simulink model "PosCtrl_tune"  (R2016b)
settings: Solver=FixedStepAuto  StartTime=0.0  StopTime=50  FixedStep=0.001  RelTol=1e-3
InitFcn:
  | Init_control;
undefined symbols (not defined in the file): DEG2RAD, DiscIntNeverNeededParam, Kd_PITCH_AgngleRate, Kd_ROLL_AgngleRate, Kd_YAW_AngleRate, Ki_PITCH_AgngleRate, Ki_ROLL_AgngleRate, Ki_YAW_AngleRate, Kp_PITCH_AgngleRate, Kp_PITCH_ANGLE, Kp_ROLL_AgngleRate, Kp_ROLL_ANGLE, Kp_YAW_AngleRate, Kpxp, Kpyp, Kpzp, Kvxd, Kvxi, Kvxp, Kvyd, Kvyi, Kvyp, Kvzd, Kvzi, Kvzp, MAX_CONTROL_ANGLE_PITCH, MAX_CONTROL_ANGLE_RATE_PITCH, MAX_CONTROL_ANGLE_RATE_ROLL, MAX_CONTROL_ANGLE_ROLL, MAX_CONTROL_VELOCITY_XY, MAX_CONTROL_VELOCITY_Z, MAX_MAN_THR, ModelInit_RPM, ModelParam_envGravityAcc, ModelParam_motorCr, ModelParam_motorJm, ModelParam_motorT, ModelParam_motorWb, ModelParam_rotorCm, ModelParam_rotorCt, ModelParam_uavCd, ModelParam_uavJ, ModelParam_uavMass, ModelParam_uavR, Saturation_I_ah, Saturation_I_az, Saturation_I_RP_Max, Saturation_I_RP_Min, Saturation_I_Y_Max, Saturation_I_Y_Min, THR_HOVER
libraries: simulink x6, aerolibutil x2, aerolibtransform2 x1
settings Model: Creator=dream  LastModifiedBy=Mr Wang
settings DebuggingCC: BusObjectLabelMismatch=error

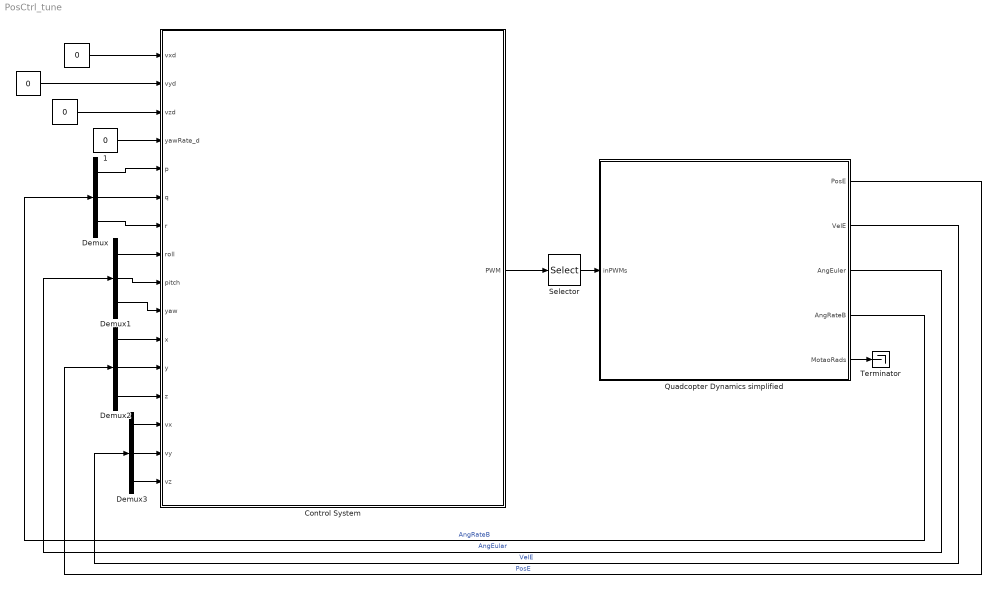
== system PosCtrl_tune ==
  "   " : Constant  Value=0  OutDataTypeStr=uint16
  "      " : Constant  Value=0  OutDataTypeStr=uint16
  "          " : Constant  Value=0  OutDataTypeStr=uint16
  "          1" : Constant  Value=0  OutDataTypeStr=uint16
  Control System : Subsystem
      mask Display: image('icon\pixhawk.png');
  Demux{,1..3} (4 alike) : Demux  Outputs=3
  "Quadcopter Dynamics simplified " : Subsystem
      mask Display: image('./icon/F450.png');
  Selector : Selector  InputPortWidth=8  IndexOptions=Index vector (dialog)  Indices=[1:4]  OutputSizes=1
  Terminator : Terminator
  wires:
  "Quadcopter Dynamics simplified "/1(PosE) -> Demux2/1  "PosE"
  "Quadcopter Dynamics simplified "/3(AngEuler) -> Demux1/1  "AngEular"
  "Quadcopter Dynamics simplified "/4(AngRateB) -> Demux/1  "AngRateB"
  Demux/1 -> Control System/5(p)
  Demux/2 -> Control System/6(q)
  Demux/3 -> Control System/7(r)
  Demux1/1 -> Control System/8(roll)
  Demux1/2 -> Control System/9(pitch)
  Demux1/3 -> Control System/10(yaw)
  Demux2/1 -> Control System/11(x)
  Demux2/2 -> Control System/12(y)
  Demux2/3 -> Control System/13(z)
  Demux3/1 -> Control System/14(vx)
  Demux3/2 -> Control System/15(vy)
  Demux3/3 -> Control System/16(vz)
  "Quadcopter Dynamics simplified "/2(VelE) -> Demux3/1  "VelE"
  "          "/1 -> Control System/3(vzd)
  "      "/1 -> Control System/2(vyd)
  "   "/1 -> Control System/1(vxd)
  "          1"/1 -> Control System/4(yawRate_d)
  Control System/1(PWM) -> Selector/1
  Selector/1 -> "Quadcopter Dynamics simplified "/1(inPWMs)
  "Quadcopter Dynamics simplified "/5(MotaoRads) -> Terminator/1

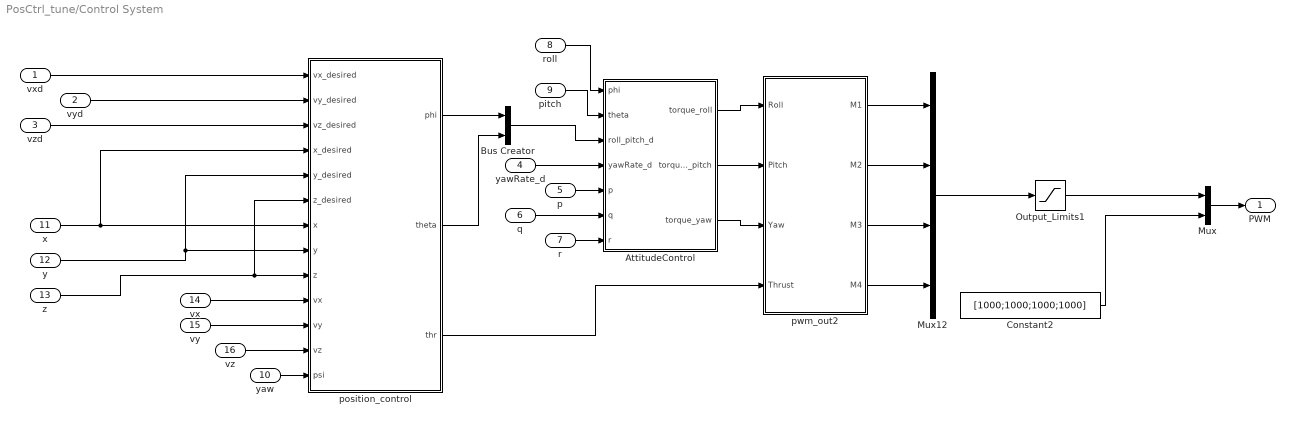
== system PosCtrl_tune/Control System ==
  vxd : Inport
  vyd : Inport  Port=2
  vzd : Inport  Port=3
  yawRate_d : Inport  Port=4
  p : Inport  Port=5  PortDimensions=1
  q : Inport  Port=6  PortDimensions=1
  r : Inport  Port=7  PortDimensions=1
  roll : Inport  Port=8  PortDimensions=1
  pitch : Inport  Port=9  PortDimensions=1
  yaw : Inport  Port=10  PortDimensions=1
  x : Inport  Port=11
  y : Inport  Port=12
  z : Inport  Port=13
  vx : Inport  Port=14
  vy : Inport  Port=15
  vz : Inport  Port=16
  AttitudeControl : Subsystem
  Bus Creator : BusCreator  Inputs=2
  Constant2 : Constant  Value=[1000;1000;1000;1000]
  Mux : Mux  Inputs=2
  Mux12 : Mux
  Output_Limits1 : Saturate  UpperLimit=2000  LowerLimit=1000
  position_control : Subsystem
  pwm_out2 : MATLAB Function  SystemSampleTime=0.004
  PWM : Outport  PortDimensions=8
  wires:
  Mux12/1 -> Output_Limits1/1
  AttitudeControl/2(torque_pitch) -> pwm_out2/2(Pitch)
  AttitudeControl/1(torque_roll) -> pwm_out2/1(Roll)
  pwm_out2/1(M1) -> Mux12/1
  pwm_out2/3(M3) -> Mux12/3
  pwm_out2/2(M2) -> Mux12/2
  AttitudeControl/3(torque_yaw) -> pwm_out2/3(Yaw)
  yawRate_d/1 -> AttitudeControl/4(yawRate_d)
  p/1 -> AttitudeControl/5(p)
  pwm_out2/4(M4) -> Mux12/4
  roll/1 -> AttitudeControl/1(phi)
  pitch/1 -> AttitudeControl/2(theta)
  position_control/1(phi) -> Bus Creator/1
  position_control/2(theta) -> Bus Creator/2
  Bus Creator/1 -> AttitudeControl/3(roll_pitch_d)
  position_control/3(thr) -> pwm_out2/4(Thrust)
  vxd/1 -> position_control/1(vx_desired)
  vyd/1 -> position_control/2(vy_desired)
  vzd/1 -> position_control/3(vz_desired)
  x/1 -> position_control/4(x_desired), position_control/7(x)
  y/1 -> position_control/5(y_desired), position_control/8(y)
  z/1 -> position_control/9(z), position_control/6(z_desired)
  vx/1 -> position_control/10(vx)
  vy/1 -> position_control/11(vy)
  vz/1 -> position_control/12(vz)
  yaw/1 -> position_control/13(psi)
  Constant2/1 -> Mux/2
  Output_Limits1/1 -> Mux/1
  Mux/1 -> PWM/1
  r/1 -> AttitudeControl/7(r)
  q/1 -> AttitudeControl/6(q)

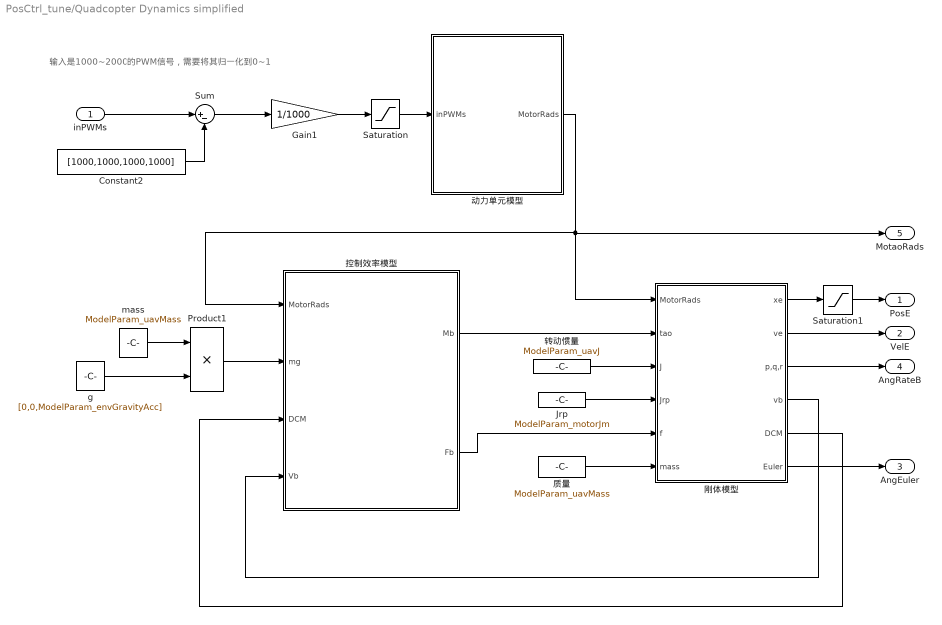
== system PosCtrl_tune/Quadcopter Dynamics simplified  ==
  note: 输入是1000~2000的PWM信号，需要将其归一化到0~1
  inPWMs : Inport
  Constant2 : Constant  Value=[1000,1000,1000,1000]
  Gain1 : Gain  Gain=1/1000
  Jrp : Constant  Value=ModelParam_motorJm
  Product1 : Product
  Saturation : Saturate  UpperLimit=1  LowerLimit=0
  Saturation1 : Saturate  UpperLimit=[inf,inf,0]  LowerLimit=[-inf,-inf,-inf]
  Sum : Sum  Inputs=|+-
  g : Constant  Value=[0,0,ModelParam_envGravityAcc]
  mass : Constant  Value=ModelParam_uavMass
  刚体模型 : Subsystem
  动力单元模型 : Subsystem
  控制效率模型 : Subsystem
  质量 : Constant  Value=ModelParam_uavMass
  转动惯量 : Constant  Value=ModelParam_uavJ
  PosE : Outport
  VelE : Outport  Port=2
  AngEuler : Outport  Port=3
  AngRateB : Outport  Port=4
  MotaoRads : Outport  Port=5
  wires:
  Saturation/1 -> 动力单元模型/1(inPWMs)
  刚体模型/3("p,q,r ") -> AngRateB/1
  Jrp/1 -> 刚体模型/4(Jrp)
  质量/1 -> 刚体模型/6(mass)
  mass/1 -> Product1/1
  刚体模型/5(DCM) -> 控制效率模型/3(DCM)
  刚体模型/1("xe ") -> Saturation1/1
  动力单元模型/1(MotorRads) -> 控制效率模型/1(MotorRads), 刚体模型/1(MotorRads), MotaoRads/1
  转动惯量/1 -> 刚体模型/3(J)
  Gain1/1 -> Saturation/1
  刚体模型/2(ve) -> VelE/1
  Sum/1 -> Gain1/1
  Product1/1 -> 控制效率模型/2(mg)
  刚体模型/4("vb ") -> 控制效率模型/4(Vb)
  Saturation1/1 -> PosE/1
  刚体模型/6(Euler) -> AngEuler/1
  控制效率模型/1(Mb) -> 刚体模型/2(tao)
  inPWMs/1 -> Sum/1
  控制效率模型/2(Fb) -> 刚体模型/5(f)
  Constant2/1 -> Sum/2
  g/1 -> Product1/2

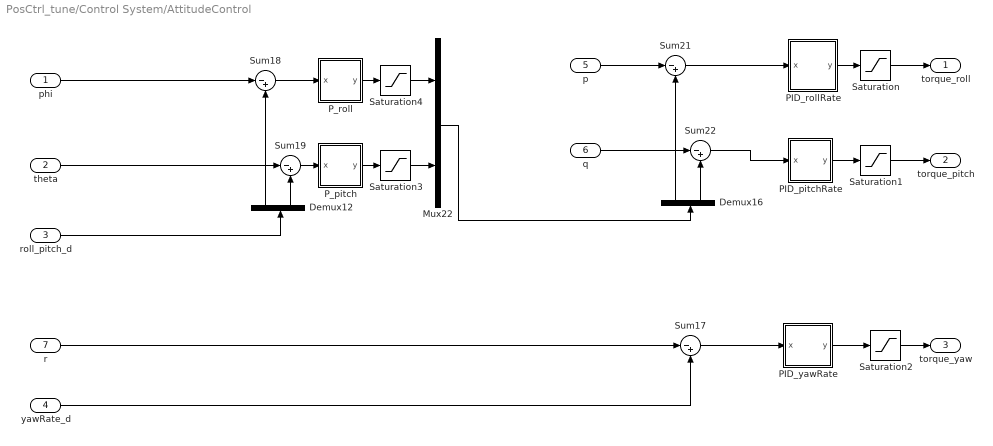
== system PosCtrl_tune/Control System/AttitudeControl ==
  phi : Inport
  theta : Inport  Port=2
  roll_pitch_d : Inport  Port=3
  yawRate_d : Inport  Port=4
  p : Inport  Port=5
  q : Inport  Port=6
  r : Inport  Port=7
  Demux12 : Demux  Outputs=2
  Demux16 : Demux  Outputs=2
  Mux22 : Mux  Inputs=2
  PID_pitchRate : Subsystem
  PID_rollRate : Subsystem
  PID_yawRate : Subsystem
  "P_pitch " : Subsystem
  "P_roll " : Subsystem
  Saturation : Saturate  UpperLimit=1  LowerLimit=-1
  Saturation1 : Saturate  UpperLimit=1  LowerLimit=-1
  Saturation2 : Saturate
  Saturation3 : Saturate  UpperLimit=MAX_CONTROL_ANGLE_RATE_PITCH  LowerLimit=-MAX_CONTROL_ANGLE_RATE_PITCH
  Saturation4 : Saturate  UpperLimit=MAX_CONTROL_ANGLE_RATE_ROLL  LowerLimit=-MAX_CONTROL_ANGLE_RATE_ROLL
  Sum{17..19,21..22} (5 alike) : Sum  Inputs=|-+
  torque_roll : Outport
  torque_pitch : Outport  Port=2
  torque_yaw : Outport  Port=3
  wires:
  r/1 -> Sum17/1
  Sum19/1 -> "P_pitch "/1(x)
  "P_pitch "/1(y) -> Saturation3/1
  "P_roll "/1(y) -> Saturation4/1
  roll_pitch_d/1 -> Demux12/1
  Demux12/1 -> Sum18/2
  Demux12/2 -> Sum19/2
  phi/1 -> Sum18/1
  theta/1 -> Sum19/1
  Sum18/1 -> "P_roll "/1(x)
  Sum22/1 -> PID_pitchRate/1(x)
  Sum17/1 -> PID_yawRate/1(x)
  p/1 -> Sum21/1
  q/1 -> Sum22/1
  Sum21/1 -> PID_rollRate/1(x)
  Demux16/1 -> Sum21/2
  PID_pitchRate/1(y) -> Saturation1/1
  PID_rollRate/1(y) -> Saturation/1
  PID_yawRate/1(y) -> Saturation2/1
  yawRate_d/1 -> Sum17/2
  Saturation/1 -> torque_roll/1
  Saturation1/1 -> torque_pitch/1
  Saturation2/1 -> torque_yaw/1
  Mux22/1 -> Demux16/1
  Saturation4/1 -> Mux22/1
  Saturation3/1 -> Mux22/2
  Demux16/2 -> Sum22/2

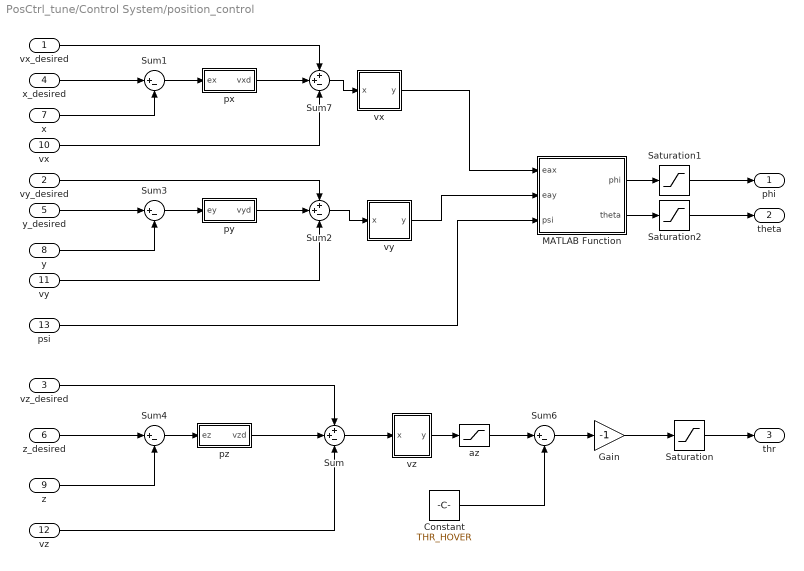
== system PosCtrl_tune/Control System/position_control ==
  vx_desired : Inport
  vy_desired : Inport  Port=2
  vz_desired : Inport  Port=3
  x_desired : Inport  Port=4
  y_desired : Inport  Port=5
  z_desired : Inport  Port=6
  x : Inport  Port=7
  y : Inport  Port=8
  z : Inport  Port=9
  vx : Inport  Port=10
  vy : Inport  Port=11
  vz : Inport  Port=12
  psi : Inport  Port=13
  Constant : Constant  Value=THR_HOVER
  Gain : Gain  Gain=-1
  MATLAB Function : MATLAB Function  TreatAsAtomicUnit=on
  Saturation : Saturate  UpperLimit=MAX_MAN_THR  LowerLimit=0
  Saturation1 : Saturate  UpperLimit=MAX_CONTROL_ANGLE_ROLL*DEG2RAD  LowerLimit=-MAX_CONTROL_ANGLE_ROLL*DEG2RAD
  Saturation2 : Saturate  UpperLimit=MAX_CONTROL_ANGLE_PITCH*DEG2RAD  LowerLimit=-MAX_CONTROL_ANGLE_PITCH*DEG2RAD
  Sum : Sum  Inputs=++-
  Sum{1,3..4,6} (4 alike) : Sum  Inputs=|+-
  Sum2 : Sum  Inputs=++-
  Sum7 : Sum  Inputs=++-
  az : Saturate  UpperLimit=0.4  LowerLimit=-0.4
  px : Subsystem
  py : Subsystem
  pz : Subsystem
  "vx " : Subsystem
  "vy " : Subsystem
  "vz " : Subsystem
  phi : Outport
  theta : Outport  Port=2
  thr : Outport  Port=3
  wires:
  Saturation/1 -> thr/1
  Gain/1 -> Saturation/1
  Sum6/1 -> Gain/1
  "vz "/1(y) -> az/1
  Sum4/1 -> pz/1(ez)
  z/1 -> Sum4/2
  Constant/1 -> Sum6/2
  Sum/1 -> "vz "/1(x)
  vz/1 -> Sum/3
  x/1 -> Sum1/2
  y/1 -> Sum3/2
  Sum3/1 -> py/1(ey)
  y_desired/1 -> Sum3/1
  vy/1 -> Sum2/3
  Sum2/1 -> "vy "/1(x)
  Sum7/1 -> "vx "/1(x)
  Sum1/1 -> px/1(ex)
  vy_desired/1 -> Sum2/1
  pz/1(vzd) -> Sum/2
  z_desired/1 -> Sum4/1
  vz_desired/1 -> Sum/1
  Saturation1/1 -> phi/1
  Saturation2/1 -> theta/1
  psi/1 -> MATLAB Function/3(psi)
  py/1(vyd) -> Sum2/2
  MATLAB Function/1(phi) -> Saturation1/1
  MATLAB Function/2(theta) -> Saturation2/1
  "vx "/1(y) -> MATLAB Function/1(eax)
  "vy "/1(y) -> MATLAB Function/2(eay)
  az/1 -> Sum6/1
  vx_desired/1 -> Sum7/1
  x_desired/1 -> Sum1/1
  vx/1 -> Sum7/3
  px/1(vxd) -> Sum7/2

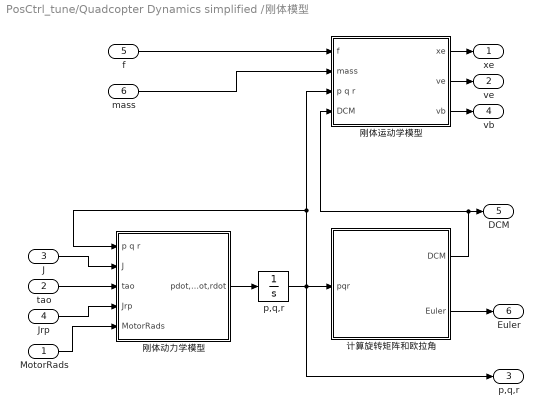
== system PosCtrl_tune/Quadcopter Dynamics simplified /刚体模型 ==
  MotorRads : Inport
  tao : Inport  Port=2
  J : Inport  Port=3
  Jrp : Inport  Port=4
  f : Inport  Port=5
  mass : Inport  Port=6
  p,q,r : Integrator
  刚体动力学模型 : Subsystem
  刚体运动学模型 : Subsystem
  计算旋转矩阵和欧拉角 : Subsystem
  "xe " : Outport
  ve : Outport  Port=2
  "p,q,r " : Outport  Port=3
  "vb " : Outport  Port=4
  DCM : Outport  Port=5
  Euler : Outport  Port=6
  wires:
  刚体运动学模型/3("vb ") -> "vb "/1
  p,q,r/1 -> 计算旋转矩阵和欧拉角/1(pqr), "p,q,r "/1, 刚体动力学模型/1(p q r), 刚体运动学模型/3(p q r)
  刚体运动学模型/2(ve) -> ve/1
  刚体运动学模型/1("xe ") -> "xe "/1
  mass/1 -> 刚体运动学模型/2(mass)
  f/1 -> 刚体运动学模型/1(f)
  计算旋转矩阵和欧拉角/2(Euler) -> Euler/1
  计算旋转矩阵和欧拉角/1(DCM) -> 刚体运动学模型/4(DCM), DCM/1
  刚体动力学模型/1(pdot,qdot,rdot) -> p,q,r/1
  MotorRads/1 -> 刚体动力学模型/5(MotorRads)
  Jrp/1 -> 刚体动力学模型/4(Jrp)
  tao/1 -> 刚体动力学模型/3(tao)
  J/1 -> 刚体动力学模型/2(J)

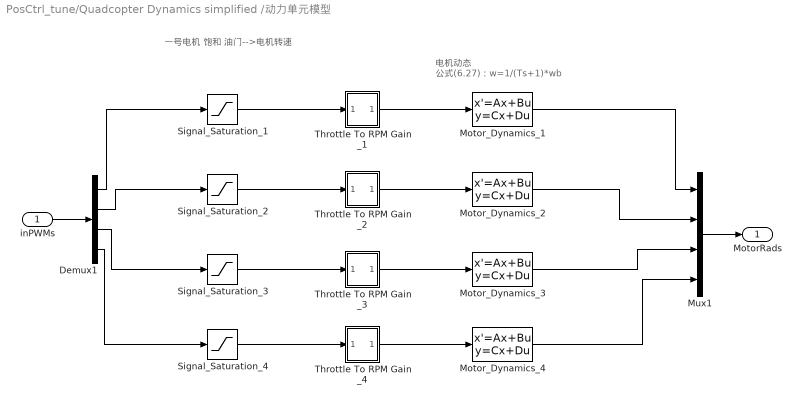
== system PosCtrl_tune/Quadcopter Dynamics simplified /动力单元模型 ==
  note: 电机动态
      | 公式(6.27)：w=1/(Ts+1)*wb
  note: 一号电机
      |
      |              饱和                             油门-->电机转速
  inPWMs : Inport
  Demux1 : Demux
  Motor_Dynamics_{1..4} (4 alike) : StateSpace  A=-1/ModelParam_motorT  C=1/ModelParam_motorT  D=0  X0=ModelInit_RPM*ModelParam_motorT
  Mux1 : Mux
  Signal_Saturation_{1..4} (4 alike) : Saturate  UpperLimit=1  LowerLimit=0
  Throttle To RPM Gain _1 : Subsystem
  Throttle To RPM Gain _2 : Subsystem
  Throttle To RPM Gain _3 : Subsystem
  Throttle To RPM Gain _4 : Subsystem
  MotorRads : Outport
  wires:
  Throttle To RPM Gain _4/1(Out5) -> Motor_Dynamics_4/1
  Signal_Saturation_4/1 -> Throttle To RPM Gain _4/1(In5)
  Signal_Saturation_3/1 -> Throttle To RPM Gain _3/1(In5)
  Signal_Saturation_2/1 -> Throttle To RPM Gain _2/1(In5)
  Motor_Dynamics_4/1 -> Mux1/4
  Motor_Dynamics_3/1 -> Mux1/3
  Motor_Dynamics_2/1 -> Mux1/2
  Motor_Dynamics_1/1 -> Mux1/1
  Signal_Saturation_1/1 -> Throttle To RPM Gain _1/1(In5)
  Mux1/1 -> MotorRads/1
  Throttle To RPM Gain _3/1(Out5) -> Motor_Dynamics_3/1
  Throttle To RPM Gain _2/1(Out5) -> Motor_Dynamics_2/1
  Throttle To RPM Gain _1/1(Out5) -> Motor_Dynamics_1/1
  inPWMs/1 -> Demux1/1
  Demux1/4 -> Signal_Saturation_4/1
  Demux1/3 -> Signal_Saturation_3/1
  Demux1/2 -> Signal_Saturation_2/1
  Demux1/1 -> Signal_Saturation_1/1

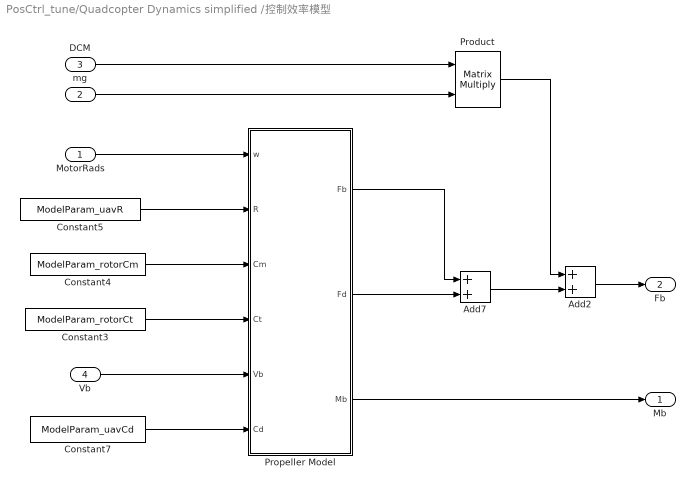
== system PosCtrl_tune/Quadcopter Dynamics simplified /控制效率模型 ==
  MotorRads : Inport
  mg : Inport  Port=2
  DCM : Inport  Port=3
  Vb : Inport  Port=4
  Add2 : Sum
  Add7 : Sum
  Constant3 : Constant  Value=ModelParam_rotorCt
  Constant4 : Constant  Value=ModelParam_rotorCm
  Constant5 : Constant  Value=ModelParam_uavR
  Constant7 : Constant  Value=ModelParam_uavCd
  Product : Product  Multiplication=Matrix(*)
  Propeller Model : MATLAB Function  TreatAsAtomicUnit=on
  Mb : Outport
  Fb : Outport  Port=2
  wires:
  Propeller Model/3(Mb) -> Mb/1
  Add2/1 -> Fb/1
  Constant3/1 -> Propeller Model/4(Ct)
  Propeller Model/2(Fd) -> Add7/2
  Add7/1 -> Add2/2
  Propeller Model/1(Fb) -> Add7/1
  Product/1 -> Add2/1
  mg/1 -> Product/2
  DCM/1 -> Product/1
  Constant7/1 -> Propeller Model/6(Cd)
  Vb/1 -> Propeller Model/5(Vb)
  Constant5/1 -> Propeller Model/2(R)
  Constant4/1 -> Propeller Model/3(Cm)
  MotorRads/1 -> Propeller Model/1(w)

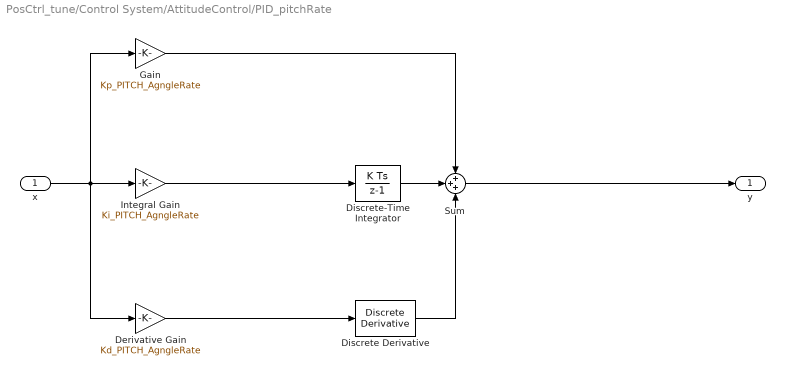
== system PosCtrl_tune/Control System/AttitudeControl/PID_pitchRate ==
  x : Inport
  Derivative Gain : Gain  DisableCoverage=on  Gain=Kd_PITCH_AgngleRate  ParamMin=-100  ParamMax=100  OutMin=-100  OutMax=100
  Discrete Derivative : simulink/Discrete/Discrete Derivative  gainval=1.0  ICPrevScaledInput=0.0  OutMin=[]  OutMax=[]  OutDataType=fixdt(1, 16)  OutScaling=2^-10  DoSatur=off
  Discrete-Time Integrator : DiscreteIntegrator  InitialConditionSetting=State (most efficient)  SampleTime=-1  LimitOutput=on  UpperSaturationLimit=Saturation_I_RP_Max  LowerSaturationLimit=Saturation_I_RP_Min  ICPrevOutput=DiscIntNeverNeededParam  ICPrevScaledInput=DiscIntNeverNeededParam
  Gain : Gain  Gain=Kp_PITCH_AgngleRate
  Integral Gain : Gain  DisableCoverage=on  Gain=Ki_PITCH_AgngleRate
  Sum : Sum  Inputs=+++
  y : Outport  InitialOutput=0
  wires:
  Discrete-Time Integrator/1 -> Sum/2
  Discrete Derivative/1 -> Sum/3
  Sum/1 -> y/1
  Gain/1 -> Sum/1
  Derivative Gain/1 -> Discrete Derivative/1
  Integral Gain/1 -> Discrete-Time Integrator/1
  x/1 -> Derivative Gain/1, Integral Gain/1, Gain/1

== system PosCtrl_tune/Control System/AttitudeControl/PID_rollRate ==
  x : Inport
  Derivative Gain : Gain  DisableCoverage=on  Gain=Kd_ROLL_AgngleRate  ParamMin=-100  ParamMax=100  OutMin=-100  OutMax=100
  Discrete Derivative : simulink/Discrete/Discrete Derivative  gainval=1.0  ICPrevScaledInput=0.0  OutMin=[]  OutMax=[]  OutDataType=fixdt(1, 16)  OutScaling=2^-10  DoSatur=off
  Discrete-Time Integrator : DiscreteIntegrator  InitialConditionSetting=State (most efficient)  SampleTime=-1  LimitOutput=on  UpperSaturationLimit=Saturation_I_RP_Max  LowerSaturationLimit=Saturation_I_RP_Min  ICPrevOutput=DiscIntNeverNeededParam  ICPrevScaledInput=DiscIntNeverNeededParam
  Gain : Gain  Gain=Kp_ROLL_AgngleRate
  Integral Gain : Gain  DisableCoverage=on  Gain=Ki_ROLL_AgngleRate
  Sum : Sum  Inputs=+++
  y : Outport  InitialOutput=0
  wires:
  x/1 -> Gain/1, Integral Gain/1, Derivative Gain/1
  Integral Gain/1 -> Discrete-Time Integrator/1
  Derivative Gain/1 -> Discrete Derivative/1
  Gain/1 -> Sum/1
  Sum/1 -> y/1
  Discrete Derivative/1 -> Sum/3
  Discrete-Time Integrator/1 -> Sum/2

== system PosCtrl_tune/Control System/AttitudeControl/PID_yawRate ==
  x : Inport
  Derivative Gain : Gain  DisableCoverage=on  Gain=Kd_YAW_AngleRate  ParamMin=-100  ParamMax=100  OutMin=-100  OutMax=100
  Discrete Derivative : simulink/Discrete/Discrete Derivative  gainval=1.0  ICPrevScaledInput=0.0  OutMin=[]  OutMax=[]  OutDataType=fixdt(1, 16)  OutScaling=2^-10  DoSatur=off
  Discrete-Time Integrator : DiscreteIntegrator  InitialConditionSetting=State (most efficient)  SampleTime=-1  LimitOutput=on  UpperSaturationLimit=Saturation_I_Y_Max  LowerSaturationLimit=Saturation_I_Y_Min  ICPrevOutput=DiscIntNeverNeededParam  ICPrevScaledInput=DiscIntNeverNeededParam
  Gain : Gain  Gain=Kp_YAW_AngleRate
  Integral Gain : Gain  DisableCoverage=on  Gain=Ki_YAW_AngleRate
  Sum : Sum  Inputs=+++
  y : Outport  InitialOutput=0
  wires:
  x/1 -> Gain/1, Integral Gain/1, Derivative Gain/1
  Integral Gain/1 -> Discrete-Time Integrator/1
  Derivative Gain/1 -> Discrete Derivative/1
  Gain/1 -> Sum/1
  Sum/1 -> y/1
  Discrete Derivative/1 -> Sum/3
  Discrete-Time Integrator/1 -> Sum/2

== system PosCtrl_tune/Control System/AttitudeControl/P_pitch  ==
  x : Inport
  Gain : Gain  Gain=Kp_PITCH_ANGLE
  y : Outport  InitialOutput=0
  wires:
  x/1 -> Gain/1
  Gain/1 -> y/1

== system PosCtrl_tune/Control System/AttitudeControl/P_roll  ==
  x : Inport
  Gain : Gain  Gain=Kp_ROLL_ANGLE
  y : Outport  InitialOutput=0
  wires:
  Gain/1 -> y/1
  x/1 -> Gain/1

== system PosCtrl_tune/Control System/position_control/px ==
  ex : Inport
  Gain1 : Gain  Gain=Kpxp
  Saturation3 : Saturate  UpperLimit=MAX_CONTROL_VELOCITY_XY  LowerLimit=-MAX_CONTROL_VELOCITY_XY
  vxd : Outport
  wires:
  ex/1 -> Gain1/1
  Saturation3/1 -> vxd/1
  Gain1/1 -> Saturation3/1

== system PosCtrl_tune/Control System/position_control/py ==
  ey : Inport
  Gain1 : Gain  Gain=Kpyp
  Saturation3 : Saturate  UpperLimit=MAX_CONTROL_VELOCITY_XY  LowerLimit=-MAX_CONTROL_VELOCITY_XY
  vyd : Outport
  wires:
  Gain1/1 -> Saturation3/1
  Saturation3/1 -> vyd/1
  ey/1 -> Gain1/1

== system PosCtrl_tune/Control System/position_control/pz ==
  ez : Inport
  Gain1 : Gain  Gain=Kpzp
  Saturation3 : Saturate  UpperLimit=MAX_CONTROL_VELOCITY_Z  LowerLimit=-MAX_CONTROL_VELOCITY_Z
  vzd : Outport
  wires:
  ez/1 -> Gain1/1
  Saturation3/1 -> vzd/1
  Gain1/1 -> Saturation3/1

== system PosCtrl_tune/Control System/position_control/vx  ==
  x : Inport
  Derivative Gain : Gain  DisableCoverage=on  Gain=Kvxd
  Discrete Derivative : simulink/Discrete/Discrete Derivative  gainval=1.0  ICPrevScaledInput=0.0  OutMin=[]  OutMax=[]  OutDataType=fixdt(1, 16)  OutScaling=2^-10  DoSatur=off
  Discrete-Time Integrator : DiscreteIntegrator  InitialConditionSetting=State (most efficient)  SampleTime=-1  LimitOutput=on  UpperSaturationLimit=Saturation_I_ah  LowerSaturationLimit=-Saturation_I_ah  ICPrevOutput=DiscIntNeverNeededParam  ICPrevScaledInput=DiscIntNeverNeededParam
  Gain : Gain  Gain=Kvxp
  Integral Gain : Gain  DisableCoverage=on  Gain=Kvxi
  Sum : Sum  Inputs=+++
  y : Outport  InitialOutput=0
  wires:
  x/1 -> Gain/1, Integral Gain/1, Derivative Gain/1
  Integral Gain/1 -> Discrete-Time Integrator/1
  Derivative Gain/1 -> Discrete Derivative/1
  Gain/1 -> Sum/1
  Sum/1 -> y/1
  Discrete Derivative/1 -> Sum/3
  Discrete-Time Integrator/1 -> Sum/2

== system PosCtrl_tune/Control System/position_control/vy  ==
  x : Inport
  Derivative Gain : Gain  DisableCoverage=on  Gain=Kvyd
  Discrete Derivative : simulink/Discrete/Discrete Derivative  gainval=1.0  ICPrevScaledInput=0.0  OutMin=-5  OutMax=5  OutDataType=fixdt(1, 16)  OutScaling=2^-10  DoSatur=off
  Discrete-Time Integrator : DiscreteIntegrator  InitialConditionSetting=State (most efficient)  SampleTime=-1  LimitOutput=on  UpperSaturationLimit=Saturation_I_ah  LowerSaturationLimit=-Saturation_I_ah  ICPrevOutput=DiscIntNeverNeededParam  ICPrevScaledInput=DiscIntNeverNeededParam
  Gain : Gain  Gain=Kvyp
  Integral Gain : Gain  DisableCoverage=on  Gain=Kvyi
  Sum : Sum  Inputs=+++  OutMin=-5  OutMax=5
  y : Outport  InitialOutput=0
  wires:
  x/1 -> Gain/1, Integral Gain/1, Derivative Gain/1
  Integral Gain/1 -> Discrete-Time Integrator/1
  Derivative Gain/1 -> Discrete Derivative/1
  Gain/1 -> Sum/1
  Sum/1 -> y/1
  Discrete Derivative/1 -> Sum/3
  Discrete-Time Integrator/1 -> Sum/2

== system PosCtrl_tune/Control System/position_control/vz  ==
  x : Inport
  Derivative Gain : Gain  DisableCoverage=on  Gain=Kvzd
  Discrete Derivative : simulink/Discrete/Discrete Derivative  gainval=1.0  ICPrevScaledInput=0.0  OutMin=[]  OutMax=[]  OutDataType=fixdt(1, 16)  OutScaling=2^-10  DoSatur=off
  Discrete-Time Integrator : DiscreteIntegrator  InitialConditionSetting=State (most efficient)  SampleTime=-1  LimitOutput=on  UpperSaturationLimit=Saturation_I_az  LowerSaturationLimit=-Saturation_I_az  ICPrevOutput=DiscIntNeverNeededParam  ICPrevScaledInput=DiscIntNeverNeededParam
  Gain : Gain  Gain=Kvzp
  Integral Gain : Gain  DisableCoverage=on  Gain=Kvzi
  Sum : Sum  Inputs=+++
  y : Outport  InitialOutput=0
  wires:
  Discrete-Time Integrator/1 -> Sum/2
  Discrete Derivative/1 -> Sum/3
  Sum/1 -> y/1
  Gain/1 -> Sum/1
  Derivative Gain/1 -> Discrete Derivative/1
  Integral Gain/1 -> Discrete-Time Integrator/1
  x/1 -> Derivative Gain/1, Integral Gain/1, Gain/1

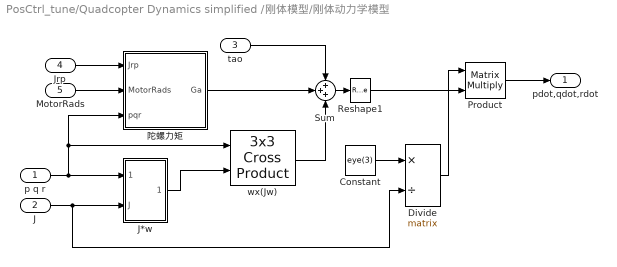
== system PosCtrl_tune/Quadcopter Dynamics simplified /刚体模型/刚体动力学模型 ==
  p q r : Inport
  J : Inport  Port=2
  tao : Inport  Port=3
  Jrp : Inport  Port=4
  MotorRads : Inport  Port=5
  Constant : Constant  Value=eye(3)
  Divide : Product  Inputs=*/  Multiplication=Matrix(*)
  J*w : Subsystem
  Product : Product  Multiplication=Matrix(*)
  Reshape1 : Reshape  OutputDimensionality=Column vector (2-D)
  Sum : Sum  Inputs=3
  wx(Jw) : aerolibutil/3x3 Cross Product
  陀螺力矩 : MATLAB Function  TreatAsAtomicUnit=on
  pdot,qdot,rdot : Outport
  wires:
  Product/1 -> pdot,qdot,rdot/1
  Reshape1/1 -> Product/2
  Constant/1 -> Divide/1
  陀螺力矩/1(Ga) -> Sum/2
  Divide/1 -> Product/1
  Sum/1 -> Reshape1/1
  J/1 -> Divide/2, J*w/2(J)
  p q r/1 -> J*w/1(p q r), 陀螺力矩/3(pqr), wx(Jw)/1
  J*w/1("J*w ") -> wx(Jw)/2
  tao/1 -> Sum/1
  Jrp/1 -> 陀螺力矩/1(Jrp)
  MotorRads/1 -> 陀螺力矩/2(MotorRads)
  wx(Jw)/1 -> Sum/3

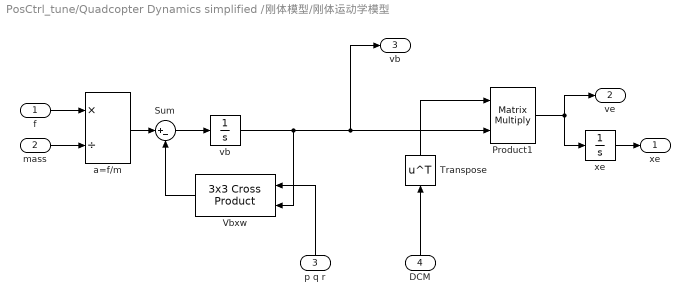
== system PosCtrl_tune/Quadcopter Dynamics simplified /刚体模型/刚体运动学模型 ==
  f : Inport
  mass : Inport  Port=2
  p q r : Inport  Port=3
  DCM : Inport  Port=4
  Product1 : Product  Multiplication=Matrix(*)
  Sum : Sum  Inputs=|+-
  Transpose : Math  Operator=transpose  SaturateOnIntegerOverflow=on
  Vbxw : aerolibutil/3x3 Cross Product
  a=f/m : Product  Inputs=*/
  vb : Integrator
  xe : Integrator
  "xe " : Outport
  ve : Outport  Port=2
  "vb " : Outport  Port=3
  wires:
  vb/1 -> Product1/2, "vb "/1, Vbxw/2
  a=f/m/1 -> Sum/1
  Sum/1 -> vb/1
  xe/1 -> "xe "/1
  Product1/1 -> xe/1, ve/1
  Transpose/1 -> Product1/1
  mass/1 -> a=f/m/2
  Vbxw/1 -> Sum/2
  f/1 -> a=f/m/1
  p q r/1 -> Vbxw/1
  DCM/1 -> Transpose/1

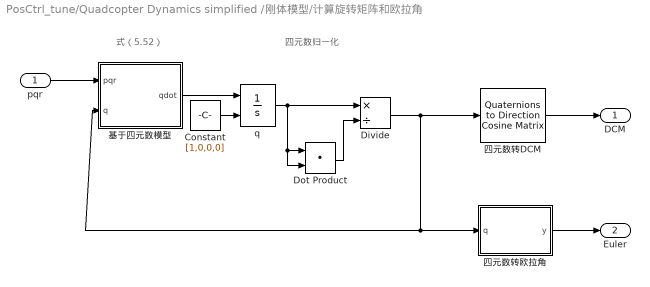
== system PosCtrl_tune/Quadcopter Dynamics simplified /刚体模型/计算旋转矩阵和欧拉角 ==
  note: 式（5.52）
  note: 四元数归一化
  pqr : Inport
  Constant : Constant  Value=[1,0,0,0]
  Divide : Product  Inputs=*/
  Dot Product : DotProduct  InputSameDT=on  OutDataTypeStr=Inherit: Inherit via internal rule
  q : Integrator  InitialConditionSource=external
  四元数转DCM : aerolibtransform2/Quaternions to  Direction Cosine Matrix
  四元数转欧拉角 : MATLAB Function
  基于四元数模型 : MATLAB Function  TreatAsAtomicUnit=on
  DCM : Outport
  Euler : Outport  Port=2
  wires:
  四元数转欧拉角/1(y) -> Euler/1
  Divide/1 -> 四元数转DCM/1, 基于四元数模型/2(q), 四元数转欧拉角/1(q)
  Dot Product/1 -> Divide/2
  四元数转DCM/1 -> DCM/1
  pqr/1 -> 基于四元数模型/1(pqr)
  q/1 -> Dot Product/1, Dot Product/2, Divide/1
  基于四元数模型/1(qdot) -> q/1
  Constant/1 -> q/2

== system PosCtrl_tune/Quadcopter Dynamics simplified /动力单元模型/Throttle To RPM Gain _1 ==
  In5 : Inport
  Constant : Constant  Value=ModelParam_motorWb
  Gain : Gain  Gain=ModelParam_motorCr
  Sum1 : Sum  Inputs=++|
  Out5 : Outport
  wires:
  Constant/1 -> Sum1/1
  Gain/1 -> Sum1/2
  In5/1 -> Gain/1
  Sum1/1 -> Out5/1

== system PosCtrl_tune/Quadcopter Dynamics simplified /动力单元模型/Throttle To RPM Gain _2 ==
  In5 : Inport
  Constant : Constant  Value=ModelParam_motorWb
  Gain : Gain  Gain=ModelParam_motorCr
  Sum1 : Sum  Inputs=++|
  Out5 : Outport
  wires:
  Sum1/1 -> Out5/1
  In5/1 -> Gain/1
  Gain/1 -> Sum1/2
  Constant/1 -> Sum1/1

== system PosCtrl_tune/Quadcopter Dynamics simplified /动力单元模型/Throttle To RPM Gain _3 ==
  In5 : Inport
  Constant : Constant  Value=ModelParam_motorWb
  Gain : Gain  Gain=ModelParam_motorCr
  Sum1 : Sum  Inputs=++|
  Out5 : Outport
  wires:
  Constant/1 -> Sum1/1
  Gain/1 -> Sum1/2
  In5/1 -> Gain/1
  Sum1/1 -> Out5/1

== system PosCtrl_tune/Quadcopter Dynamics simplified /动力单元模型/Throttle To RPM Gain _4 ==
  In5 : Inport
  Constant : Constant  Value=ModelParam_motorWb
  Gain : Gain  Gain=ModelParam_motorCr
  Sum1 : Sum  Inputs=++|
  Out5 : Outport
  wires:
  Sum1/1 -> Out5/1
  In5/1 -> Gain/1
  Gain/1 -> Sum1/2
  Constant/1 -> Sum1/1

== system PosCtrl_tune/Quadcopter Dynamics simplified /刚体模型/刚体动力学模型/J*w ==
  p q r : Inport
  J : Inport  Port=2
  J*w : Product  Multiplication=Matrix(*)
  "J*w " : Outport
  wires:
  J*w/1 -> "J*w "/1
  J/1 -> J*w/1
  p q r/1 -> J*w/2

== matlab function PosCtrl_tune/Control System/position_control/MATLAB Function ==
  data: eax input; eay input; psi input; phi output; theta output
function [phi,theta] = fcn(eax,eay,psi)
g=9.8;
phi = (-sin(psi)*eax + cos(psi)*eay)/g;
theta = (-cos(psi)*eax-sin(psi)*eay)/g;

== matlab function PosCtrl_tune/Control System/pwm_out2 ==
  data: Roll input; M1 output; Pitch input; Yaw input; Thrust input; M2 output; M3 output; M4 output
function [M1, M2, M3, M4] = motor_mixer(Roll, Pitch, Yaw, Thrust)
%quadrotorX
%3     1
%  \ /
%  / \
%2     4

idle_PWM = 1000;
scale = 1000;

M1 = (Thrust - Roll + Pitch + Yaw) * scale + idle_PWM;
M2 = (Thrust + Roll - Pitch + Yaw) * scale + idle_PWM;
M3 = (Thrust + Roll + Pitch - Yaw) * scale + idle_PWM;
M4 = (Thrust - Roll - Pitch - Yaw) * scale + idle_PWM;

== matlab function PosCtrl_tune/Quadcopter Dynamics simplified /刚体模型/刚体动力学模型/陀螺力矩 ==
  data: Jrp input; MotorRads input; pqr input; Ga output
function Ga = fcn(Jrp,MotorRads,pqr)
Ga=zeros(3,1);
Ga(1)=Jrp*pqr(2)*(-MotorRads(1)-MotorRads(2)+MotorRads(3)+MotorRads(4));
Ga(2)=Jrp*pqr(1)*( MotorRads(1)+MotorRads(2)-MotorRads(3)-MotorRads(4));

== matlab function PosCtrl_tune/Quadcopter Dynamics simplified /刚体模型/计算旋转矩阵和欧拉角/四元数转欧拉角 ==
  data: q input; y output
function y = fcn(q)
Rbe = [q(1)*q(1) + q(2)*q(2) - q(3)*q(3) - q(4)*q(4), 2*(q(2)*q(3) - q(1)*q(4)), 2*(q(2)*q(4) + q(1)*q(3))
       2*(q(2)*q(3) + q(1)*q(4)), q(1)*q(1) - q(2)*q(2) + q(3)*q(3) - q(4)*q(4), 2*(q(3)*q(4) - q(1)*q(2))
       2*(q(2)*q(4) - q(1)*q(3)), 2*(q(3)*q(4) + q(1)*q(2)), q(1)*q(1) - q(2)*q(2) - q(3)*q(3) + q(4)*q(4)];
   
phi = atan2(Rbe(3,2),Rbe(3,3));
theta = asin(-Rbe(3,1));
psi = atan2(Rbe(2,1),Rbe(1,1));  
% phi = atan2(2*(q(1)*q(2)+q(3)*q(4)),(1-2*(q(2)*q(2)+q(3)*q(3))));
% theta = asin(2*(q(1)*q(3)-q(2)*q(4)));
% psi = atan2(2*(q(1)*q(4)+q(2)*q(3)),(1-2*(q(3)*q(3))+q(4)*q(4)));
y = [phi theta psi];

== matlab function PosCtrl_tune/Quadcopter Dynamics simplified /刚体模型/计算旋转矩阵和欧拉角/基于四元数模型 ==
  data: pqr input; qdot output; q input
function qdot = fcn(pqr,q)

qdot=0.5*[0,-pqr(1),-pqr(2),-pqr(3);pqr(1),0,pqr(3),-pqr(2);pqr(2),-pqr(3),0,pqr(1);pqr(3),pqr(2),-pqr(1),0]*q;

== matlab function PosCtrl_tune/Quadcopter Dynamics simplified /控制效率模型/Propeller Model ==
  data: w input; R input; Fb output; Fd output; Mb output; Cm input; Ct input; Vb input; Cd input
function [Fb,Fd,Mb] = fcn(w,R,Cm,Ct,Vb,Cd)
 %%叉字型
 %3  1
 %2  4
 M_rctcm = [-sin(pi/4)*R*Ct,sin(pi/4)*R*Ct,sin(pi/4)*R*Ct,-sin(pi/4)*R*Ct;
            sin(pi/4)*R*Ct,-sin(pi/4)*R*Ct,sin(pi/4)*R*Ct,-sin(pi/4)*R*Ct;
            Cm,Cm,-Cm,-Cm];
 Mb = M_rctcm*(w.^2);%式(6.24),力矩
 
 Fb = [0; 0; -sum(Ct*(w.^2))]; %(6.23),螺旋桨拉力
 Fd = -Cd*Vb.*abs(Vb)*0.5;%空气阻力
end
